simulink model "test_123"  (R2022a)
settings: Solver=VariableStepAuto  StartTime=0.0  StopTime=10.0  RelTol=1e-3
settings Model: Creator=kimsd  LastModifiedBy=kimsd

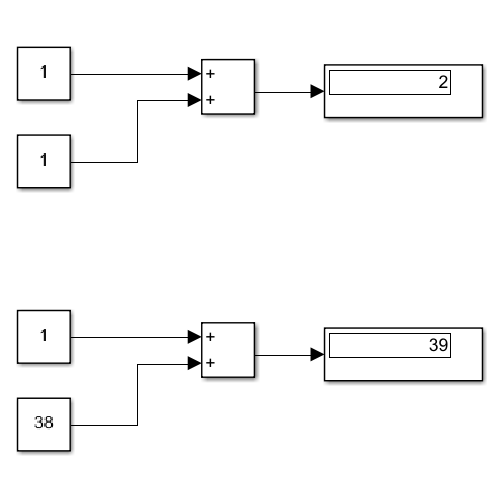
[thumbnail: Simulink's stored preview of the top-level diagram]
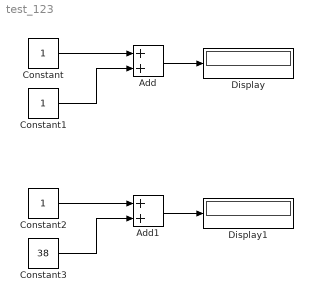
== system test_123 ==
  Add : Sum
  Add1 : Sum
  Constant : Constant
  Constant1 : Constant
  Constant2 : Constant
  Constant3 : Constant  Value=38
  Display : Display
  Display1 : Display
  wires:
  Add/1 -> Display/1
  Constant/1 -> Add/1
  Constant1/1 -> Add/2
  Constant3/1 -> Add1/2
  Constant2/1 -> Add1/1
  Add1/1 -> Display1/1
